simulink model "Actormodel"  (R2018b)
settings: Solver=VariableStepAuto  StartTime=0.0  StopTime=10.0  RelTol=1e-3
libraries: neural x904
(part 25 of 25)

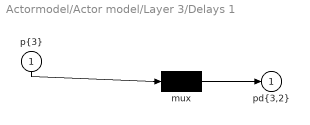
== system Actormodel/Actor model/Layer 3/Delays 1 ==
  "p{3}" : Inport  PortDimensions=600
      mask Display: e = 0.06;c1 = [120 230 180]/255;c2 = ([120 230 180]+0)/(256+128);c3 = ([120 230 180]+128)/(256+128);patch([0 1 1 0],[0 0 1 1],c1);patch([0 1 1 1-e 1-e 0+e],[0 0 1 1-e 0+e 0+e],c2);patch([0 0 1 1-e 0+e 0+e],[0 1 1 1-e 1-e 0+e],c3);plot([0 1 1 0 0],[0 0 1 1 0]);
  mux : Mux  Inputs=1
      mask Display: e = 0.06;c1 = [120 150 230]/255;c2 = ([120 150 230]+0)/383;c3 = ([120 150 230]+128)/383;patch([0 1 1 0],[0 0 1 1],c1);patch([0 1 1 1-e 1-e 0+e],[0 0 1 1-e 0+e 0+e],c2);patch([0 0 1 1-e 0+e 0+e],[0 1 1 1-e 1-e 0+e],c3);plot([0 1 1 0 0],[0 0 1 1 0]);disp('Mux')
  "pd{3,2}" : Outport
      mask Display: e = 0.06;c1 = [120 230 180]/255;c2 = ([120 230 180]+0)/(256+128);c3 = ([120 230 180]+128)/(256+128);patch([0 1 1 0],[0 0 1 1],c1);patch([0 1 1 1-e 1-e 0+e],[0 0 1 1-e 0+e 0+e],c2);patch([0 0 1 1-e 0+e 0+e],[0 1 1 1-e 1-e 0+e],c3);plot([0 1 1 0 0],[0 0 1 1 0]);
  wires:
  "p{3}"/1 -> mux/1
  mux/1 -> "pd{3,2}"/1

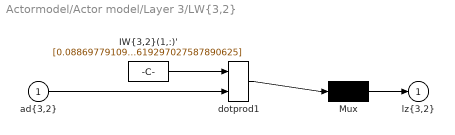
== system Actormodel/Actor model/Layer 3/LW{3,2} ==
  "ad{3,2}" : Inport  PortDimensions=600
      mask Display: e = 0.06;c1 = [120 230 180]/255;c2 = ([120 230 180]+0)/(256+128);c3 = ([120 230 180]+128)/(256+128);patch([0 1 1 0],[0 0 1 1],c1);patch([0 1 1 1-e 1-e 0+e],[0 0 1 1-e 0+e 0+e],c2);patch([0 0 1 1-e 0+e 0+e],[0 1 1 1-e 1-e 0+e],c3);plot([0 1 1 0 0],[0 0 1 1 0]);
  "IW{3,2}(1,:)'" : Constant  Value=[0.08869779109954833984375;-0.02772250212728977203369140625;0.0170603431761264801025390625;0.15445093810558319091796875;-0.20952297747135162353515625;0.14824092388153076171875;0.17191345989704132080078125;-0.0429236404597759246826171875;-0.086115010082721710205078125;0.083174161612987518310546875;0.080997250974178314208984375;0.113963879644870758056640625;0.061717510223388671875;0.20270146429538726806640625;0.22841370105743408203125;0.123978175222873687744140625;-0.122170470654964447021484375;0.09792287647724151611328125;-0.0212429352104663848876953125;-0.00431523285806179046630859375;0.13820545375347137451171875;-0.1569981276988983154296875;0.0381511189043521881103515625;0.21562124788761138916015625;-0.092364840209484100341796875;0.009731735102832317352294921875;-0.0616881512105464935302734375;-0.2106240689754486083984375;-0.0069645405746996402740478515625;-0.18533949553966522216796875;-0.13136099278926849365234375;0.02765651233494281768798828125;-0.12016476690769195556640625;0.14648117125034332275390625;0.15320615470409393310546875;0.10413633286952972412109375;-0.108559049665927886962890625;-0.1031062602996826171875;0.17941536009311676025390625;-0.3394639790058135986328125;0.080109782516956329345703125;-0.086637161672115325927734375;-0.14775933325290679931640625;-0.12505124509334564208984375;0.1442160308361053466796875;0.007784941233694553375244140625;0.090372107923030853271484375;0.12918198108673095703125;0.18843097984790802001953125;0.069990813732147216796875;-0.1445629596710205078125;0.112689547240734100341796875;-0.13051570951938629150390625;-0.1296372115612030029296875;-0.132935702800750732421875;0.028374135494232177734375;-0.15735130012035369873046875;-0.1309014260768890380859375;0.1064789295196533203125;0.120984233915805816650390625;-0.13780228793621063232421875;0.1254282891750335693359375;0.0721547305583953857421875;0.0324240140616893768310546875;0.0211966298520565032958984375;0.0403634719550609588623046875;0.081876523792743682861328125;-0.058832593262195587158203125;0.14161886274814605712890625;0.14213313162326812744140625;0.2163051068782806396484375;0.121490590274333953857421875;0.13311769068241119384765625;0.03475296497344970703125;-0.16078464686870574951171875;-0.13232590258121490478515625;-0.118817992508411407470703125;-0.16370593011379241943359375;0.12303769588470458984375;-0.0823805034160614013671875;0.078410767018795013427734375;0.075638867914676666259765625;0.118029691278934478759765625;-0.110427670180797576904296875;0.1337440907955169677734375;0.1052784621715545654296875;-0.006561194546520709991455078125;0.14115987718105316162109375;0.163374245166778564453125;0.2455030977725982666015625;0.1414764821529388427734375;0.14920617640018463134765625;0.1602183878421783447265625;0.077757306396961212158203125;0.009015818126499652862548828125;0.1279061138629913330078125;-0.1296041309833526611328125;0.11720497906208038330078125;-0.002901147119700908660888671875;0.1704672276973724365234375;0.0722072124481201171875;0.139283835887908935546875;-0.1386676728725433349609375;-0.2813821136951446533203125;0.14788998663425445556640625;-0.1542265415191650390625;-0.056217916309833526611328125;-0.02953671850264072418212890625;0.0370835363864898681640625;0.071201376616954803466796875;0.10709284245967864990234375;0.120956473052501678466796875;0.17929010093212127685546875;0.136342465877532958984375;0.154359877109527587890625;-0.010153892450034618377685546875;0.098805613815784454345703125;0.1968474686145782470703125;0.102073781192302703857421875;0.1631968319416046142578125;0.0820573270320892333984375;0.08919467031955718994140625;0.1313992440700531005859375;-0.216116428375244140625;0.28973782062530517578125;0.17866744101047515869140625;-0.1266472637653350830078125;0.000243416681769303977489471435546875;-0.0481970794498920440673828125;0.15563543140888214111328125;0.13476233184337615966796875;0.117798812687397003173828125;-0.0211709327995777130126953125;0.18279401957988739013671875;0.067768178880214691162109375 ...(+13705 chars)]
      mask Display: e = 0.06;c1 = [120 150 230]/255;c2 = ([120 150 230]+0)/383;c3 = ([120 150 230]+128)/383;patch([0 1 1 0],[0 0 1 1],c1);patch([0 1 1 1-e 1-e 0+e],[0 0 1 1-e 0+e 0+e],c2);patch([0 0 1 1-e 0+e 0+e],[0 1 1 1-e 1-e 0+e],c3);plot([0 1 1 0 0],[0 0 1 1 0]);disp('weights');
  Mux : Mux  Inputs=1
      mask Display: e = 0.06;c1 = [120 150 230]/255;c2 = ([120 150 230]+0)/383;c3 = ([120 150 230]+128)/383;patch([0 1 1 0],[0 0 1 1],c1);patch([0 1 1 1-e 1-e 0+e],[0 0 1 1-e 0+e 0+e],c2);patch([0 0 1 1-e 0+e 0+e],[0 1 1 1-e 1-e 0+e],c3);plot([0 1 1 0 0],[0 0 1 1 0]);disp('Mux');
  dotprod1 : neural/Weight Functions/dotprod
  "lz{3,2}" : Outport
      mask Display: e = 0.06;c1 = [120 230 180]/255;c2 = ([120 230 180]+0)/(256+128);c3 = ([120 230 180]+128)/(256+128);patch([0 1 1 0],[0 0 1 1],c1);patch([0 1 1 1-e 1-e 0+e],[0 0 1 1-e 0+e 0+e],c2);patch([0 0 1 1-e 0+e 0+e],[0 1 1 1-e 1-e 0+e],c3);plot([0 1 1 0 0],[0 0 1 1 0]);
  wires:
  "IW{3,2}(1,:)'"/1 -> dotprod1/1
  "ad{3,2}"/1 -> dotprod1/2
  dotprod1/1 -> Mux/1
  Mux/1 -> "lz{3,2}"/1
